simulink model "sensor_reading"  (R2024a)
settings: Solver=VariableStepAuto  StartTime=0.0  StopTime=inf  MaxStep=1e-3  MinStep=1e-5  RelTol=1e-4
InitFcn:
  | id_setup()
StartFcn:
  | c_id = evalin('base', "car_id");
  | g_id = evalin('base', "group_id");
  | mqttBasic(c_id,g_id);
libraries: read x5, uavutilslib x1, instrumentlib x1, init x1
settings Model: Creator=adriaeik  LastModifiedBy=adriaeik
settings DebuggingCC: UnderSpecifiedDimensionMsg=warning

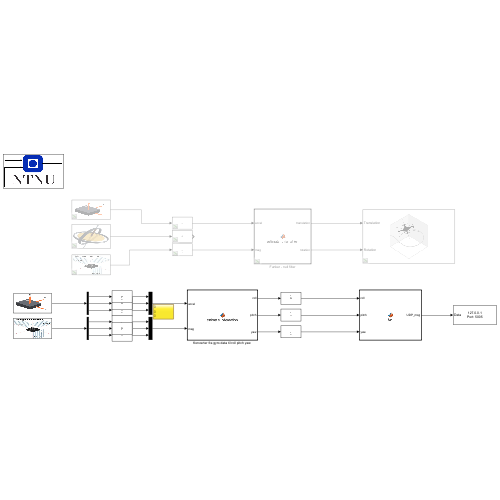
[thumbnail: Simulink's stored preview of the top-level diagram]
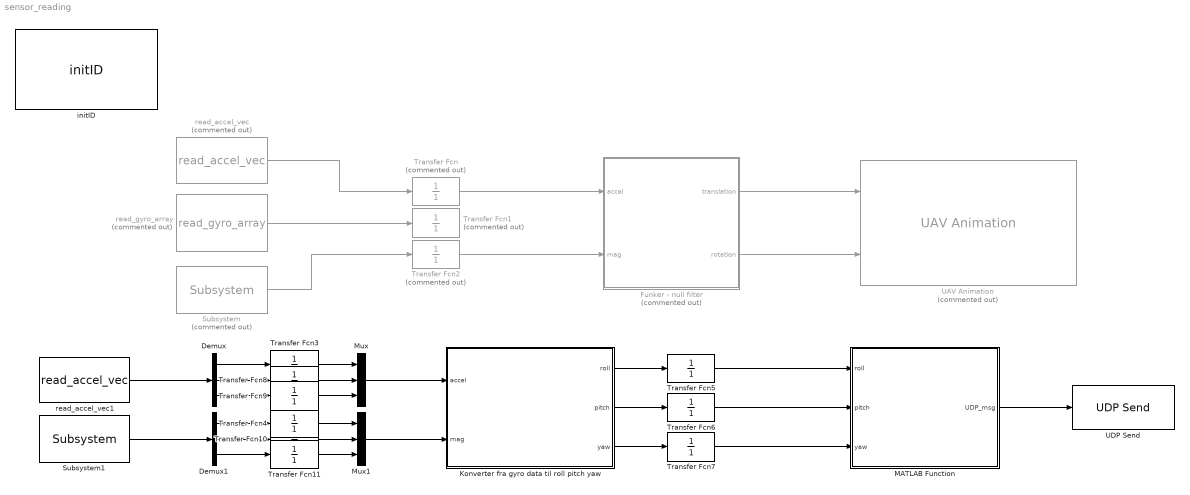
== system sensor_reading ==
  Demux : Demux  Outputs=3
  Demux1 : Demux  Outputs=3
  Funker - null filter : MATLAB Function  Commented=on  TreatAsAtomicUnit=on
  "Konverter fra gyro data til roll pitch yaw " : MATLAB Function  TreatAsAtomicUnit=on
  MATLAB Function : MATLAB Function  TreatAsAtomicUnit=on
  Mux : Mux  Inputs=3
  Mux1 : Mux  Inputs=3
  Subsystem : read/Subsystem  Commented=on
  Subsystem1 : read/Subsystem
  Transfer Fcn : TransferFcn  Commented=on  Denominator=[0 1]
  Transfer Fcn1 : TransferFcn  Commented=on  Denominator=[0 1]
  Transfer Fcn{3..11} (9 alike) : TransferFcn  Denominator=[0 1]
  Transfer Fcn2 : TransferFcn  Commented=on  Denominator=[0 1]
  UAV Animation : uavutilslib/UAV Animation  Commented=on  UAVType=Multirotor  UAVSize=1  InertialZDirection=Up  SampleTime=0.1
  UDP Send : instrumentlib/UDP Send  Host=127.0.0.1  Port=5005  LocalAddress=0.0.0.0  LocalPort=-1  EnablePortSharing=off  OutputDatagramPacketSize=8  ByteOrder=big-endian  EnableBlockingMode=on  SimulateUsing=Interpreted execution
  initID : init/initID  carID=0  groupID=0
  read_accel_vec : read/read_accel_vec  Commented=on
  read_accel_vec1 : read/read_accel_vec
  read_gyro_array : read/read_gyro_array  Commented=on
  wires:
  Subsystem/1 -> Transfer Fcn2/1
  read_accel_vec/1 -> Transfer Fcn/1
  Funker - null filter/1(translation) -> UAV Animation/1
  Funker - null filter/2(rotation) -> UAV Animation/2
  Transfer Fcn/1 -> Funker - null filter/1(accel)
  Transfer Fcn2/1 -> Funker - null filter/2(mag)
  read_gyro_array/1 -> Transfer Fcn1/1
  Mux/1 -> "Konverter fra gyro data til roll pitch yaw "/1(accel)
  read_accel_vec1/1 -> Demux/1
  Subsystem1/1 -> Demux1/1
  "Konverter fra gyro data til roll pitch yaw "/1(roll) -> Transfer Fcn5/1
  "Konverter fra gyro data til roll pitch yaw "/3(yaw) -> Transfer Fcn7/1
  "Konverter fra gyro data til roll pitch yaw "/2(pitch) -> Transfer Fcn6/1
  Transfer Fcn5/1 -> MATLAB Function/1(roll)
  Transfer Fcn6/1 -> MATLAB Function/2(pitch)
  Transfer Fcn7/1 -> MATLAB Function/3(yaw)
  MATLAB Function/1(UDP_msg) -> UDP Send/1
  Transfer Fcn9/1 -> Mux/3
  Demux/3 -> Transfer Fcn9/1
  Demux/2 -> Transfer Fcn8/1
  Demux/1 -> Transfer Fcn3/1
  Transfer Fcn3/1 -> Mux/1
  Transfer Fcn8/1 -> Mux/2
  Demux1/3 -> Transfer Fcn11/1
  Transfer Fcn11/1 -> Mux1/3
  Demux1/2 -> Transfer Fcn10/1
  Transfer Fcn10/1 -> Mux1/2
  Transfer Fcn4/1 -> Mux1/1
  Demux1/1 -> Transfer Fcn4/1
  Mux1/1 -> "Konverter fra gyro data til roll pitch yaw "/2(mag)

== matlab function sensor_reading/MATLAB Function ==
  data: roll input; pitch input; yaw input; UDP_msg output size=[8 1]
function UDP_msg = fcn(roll, pitch, yaw)

R_bw = eul2rotm([yaw, pitch, roll], 'ZYX'); 

z_vec = [0; 0; 1]; 

Rot_joystick = R_bw * z_vec; 



y = Rot_joystick(1);
x = Rot_joystick(2); 


%Ikke tenk på det
xy_single = single([x; y]);
xy_be     = swapbytes(xy_single);

UDP_msg = typecast(xy_be, 'uint8');

== matlab function sensor_reading/Konverter fra gyro data til roll pitch yaw  ==
  data: accel input; roll output; mag input; pitch output; yaw output
function [roll, pitch, yaw] = estimate_orientation(accel, mag)
%#codegen

% accel, gyro, mag: [3x1] sensorvektorar
% gyro(3) er yaw i radianar (allerede integrert)

% --- Normaliser og formater ---
accel = accel(:); accel = accel / norm(accel);
mag   = mag(:);   mag = mag / norm(mag);


% --- Estimer roll og pitch frå akselerometer ---


%%%
% Regn ut selv! 

raw_pitch = atan2(accel(1), sqrt(accel(2)^2 + accel(3)^2));
raw_roll  = atan2(-accel(2), accel(3));





%%%


% --- Tiltkompensasjon av magnetometer ---
Rx = [1 0 0;
      0 cos(raw_roll) -sin(raw_roll);
      0 sin(raw_roll)  cos(raw_roll)];
Ry = [cos(raw_pitch) 0 sin(raw_pitch);
      0 1 0;
     -sin(raw_pitch) 0 cos(raw_pitch)];

R = Ry * Rx;
mag_flat = R' * mag;  % kompenser for tilt
raw_yaw = atan2(-mag_flat(2), mag_flat(1));


roll = raw_roll; 
pitch = raw_pitch; 
yaw = raw_yaw;

== matlab function sensor_reading/Funker - null filter ==
  settings: updateMethod=DISCRETE
  data: accel input; translation output; mag input; rotation output
function [translation, rotation] = estimate_orientation(accel, mag)
%#codegen

% accel, gyro, mag: [3x1] sensorvektorar
% gyro(3) er yaw i radianar (allerede integrert)

% --- Normaliser og formater ---
accel = accel(:); accel = accel / norm(accel);
mag   = mag(:);   mag = mag / norm(mag);

% --- Persistent for filtering ---
persistent last_pitch last_roll last_yaw
if isempty(last_pitch)
    last_pitch = 0; last_roll = 0; last_yaw = atan2(-accel(2), accel(3));
end

% --- Estimer roll og pitch frå akselerometer ---
raw_pitch = atan2(accel(1), sqrt(accel(2)^2 + accel(3)^2));
raw_roll  = atan2(-accel(2), accel(3));







% --- Tiltkompensasjon av magnetometer ---
Rx = [1 0 0;
      0 cos(raw_roll) -sin(raw_roll);
      0 sin(raw_roll)  cos(raw_roll)];
Ry = [cos(raw_pitch) 0 sin(raw_pitch);
      0 1 0;
     -sin(raw_pitch) 0 cos(raw_pitch)];

R = Ry * Rx;
mag_flat = R' * mag;  % kompenser for tilt

% --- Estimer yaw frå mag (valgfritt, for driftkompensasjon) ---
raw_yaw = atan2(-mag_flat(2), mag_flat(1));  % N = 0 rad


% --- Lavpassfilter Euler-vinklar ---
beta = 0.95;
pitch = beta * last_pitch + (1 - beta) * raw_pitch;
roll  = beta * last_roll  + (1 - beta) * raw_roll;
yaw   = beta * last_yaw   + (1 - beta) * raw_yaw;

last_pitch = pitch;
last_roll  = roll;
last_yaw   = yaw;

% --- Konverter Euler til kvaternion [w x y z] ---
q = eul2quat([yaw, pitch, roll], 'ZYX');
rotation = q(:);

% Dummy posisjon
translation = [0; 0; 0];
end
